simulink model "tasten_model"  (R2021b)
settings: Solver=ode4  StartTime=0.0  StopTime=30  FixedStep=0.01  RelTol=1e-3
values from neighbouring files (symbols this model uses):
  k = 1.2    [tasten.m]
  k1 = 0.28    [tasten.m]
  k2 = 1.5    [tasten.m]
  tau = 0.5    [tasten.m]
settings Model: Creator=dmitr  LastModifiedBy=dmitr

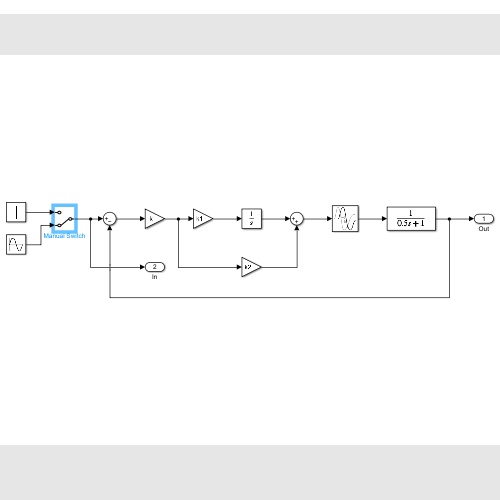
[thumbnail: Simulink's stored preview of the top-level diagram]
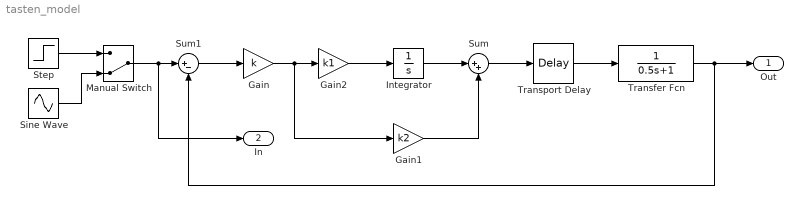
== system tasten_model ==
  Gain : Gain  Gain=k
  Gain1 : Gain  Gain=k2
  Gain2 : Gain  Gain=k1
  Integrator : Integrator
  Manual Switch : ManualSwitch  CurrentSetting=0
  Sine Wave : Sin  SampleTime=0
  Step : Step  Time=0  SampleTime=0
  Sum : Sum  Inputs=|++
  Sum1 : Sum  Inputs=|+-
  Transfer Fcn : TransferFcn  Denominator=[0.5 1]
  Transport Delay : TransportDelay  DelayTime=tau
  Out : Outport
  In : Outport  Port=2
  wires:
  Gain/1 -> Gain2/1, Gain1/1
  Integrator/1 -> Sum/1
  Gain1/1 -> Sum/2
  Sum1/1 -> Gain/1
  Sum/1 -> Transport Delay/1
  Transport Delay/1 -> Transfer Fcn/1
  Transfer Fcn/1 -> Out/1, Sum1/2
  Gain2/1 -> Integrator/1
  Step/1 -> Manual Switch/1
  Manual Switch/1 -> In/1, Sum1/1
  Sine Wave/1 -> Manual Switch/2
